simulink model "regulator_LQG_discrete_Ueq_comparison"  (R2019b)
settings: Solver=ode45  StartTime=0.0  StopTime=tsim  RelTol=1e-3  EnableMultiTasking=on
values from neighbouring files (symbols this model uses):
  B_noise = [B ones(size(B,1),1)]    [es3.m]
  C_states = eye(2)    [es3.m]
  D_noise = [D_states zeros(size(D_states,1),1)]    [es3.m]
  Klqr1 = dlqr(A,B,Q,R)    [es3.m]
  NK = 0    [es3.m]
  RK1 = 10*QK(1)    [es3.m]
  RK2 = QK(1)*0.1    [es3.m]
  sat_max = inf    [es3.m]
  sat_min = -inf    [es3.m]
  Ts = 0.1    [es3.m]
  Ubar = inv(dcgain(Gz))*Ybar    [es3.m]
  x0 = [5 20]    [es3.m]
  x0K = 1.5*x0    [es3.m]
  xref = Xbar    [es3.m]
undefined symbols (not defined in the file or in its folder): A, B, C, D, Discrete, Time
libraries: simulink x4, ctrlSharedLib x2
settings Model: Creator=Administrator  LastModifiedBy=Chiara
settings DataIOCC: LimitDataPoints=on  SaveFormat=Array  SignalLoggingSaveFormat=ModelDataLogs  ReturnWorkspaceOutputs=off
settings OptimizationCC: ExpressionDepthLimit=2147483647  InitFltsAndDblsToZero=on  LifeSpan=inf
settings DebuggingCC: UnderspecifiedInitializationDetection=Classic  MergeDetectMultiDrivingBlocksExec=none  SolverPrmCheckMsg=warning  FcnCallInpInsideContextMsg=warning  StateNameClashWarn=warning  SFUnexpectedBacktrackingDiag=warning  SFNoUnconditionalDefaultTransitionDiag=warning  SFExecutionAtInitializationDiag=none  ArithmeticOperatorsInVariantConditions=warning
settings HardwareCC: ProdBitPerPointer=32  ProdBitPerSizeT=32  ProdBitPerPtrDiffT=32  ProdLargestAtomicFloat=None  ProdIntDivRoundTo=Undefined  ProdEndianess=Unspecified  ProdWordSize=32  ProdHWDeviceType=32-bit Generic
settings ModelReferenceCC: PropagateSignalLabelsOutOfModel=off
settings SFSimCC: SimUseLocalCustomCode=off  CustomCodeUndefinedFunction=UseInterfaceOnly
settings RTWCC: RTWUseLocalCustomCode=off
settings CodeAppCC: StateflowObjectComments=on
settings GRTTargetCC: TargetLangStandard=C89/C90 (ANSI)  GeneratePreprocessorConditionals=Disable all  CombineOutputUpdateFcns=off  GRTInterface=on
settings ConfigComp: CovMetricSettings=dw  CovHtmlReporting=on  CovSaveCumulativeToWorkspaceVar=on  CovSaveSingleToWorkspaceVar=on  CovExternalEMLEnable=off  CovSFcnEnable=off

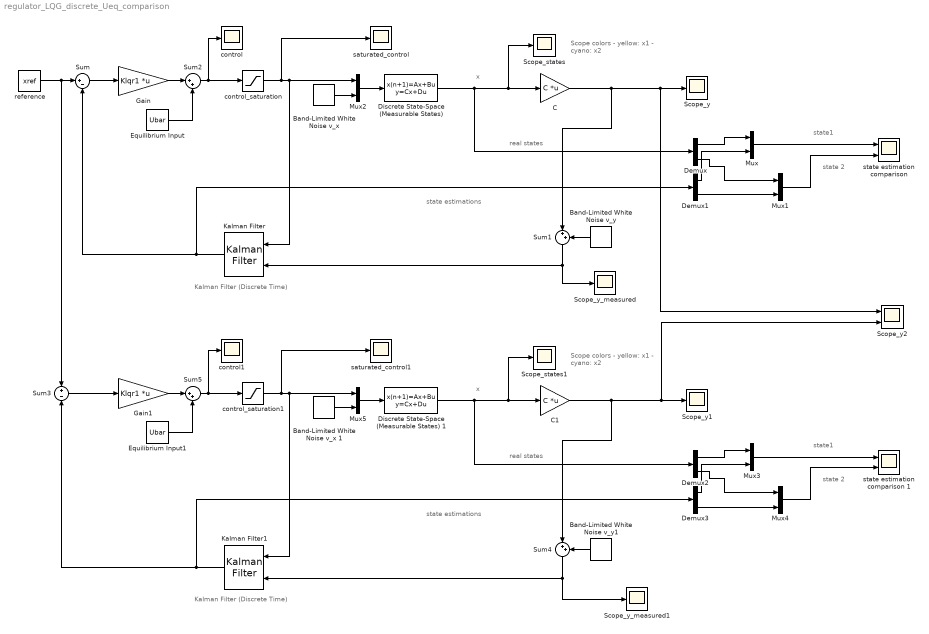
== system regulator_LQG_discrete_Ueq_comparison ==
  note: Kalman Filter (Discrete Time)
  note: state 2
  note: state1
  note: real states
  note: state estimations
  note: x
  note: Scope colors
      | - yellow: x1
      | - cyano: x2
  note: x
  note: state 2
  note: Scope colors
      | - yellow: x1
      | - cyano: x2
  note: Kalman Filter (Discrete Time)
  note: real states
  note: state1
  note: state estimations
  "Band-Limited White Noise v_x " : simulink/Sources/Band-Limited White Noise  Cov=power_vx1  Ts=Ts  seed=[23341]
  Band-Limited White Noise v_x 1 : simulink/Sources/Band-Limited White Noise  Cov=power_vx2  Ts=Ts  seed=[23341]
  Band-Limited White Noise v_y : simulink/Sources/Band-Limited White Noise  Cov=power_vy1  Ts=Ts  seed=[1258]
  Band-Limited White Noise v_y1 : simulink/Sources/Band-Limited White Noise  Cov=power_vy2  Ts=Ts  seed=[1258]
  C : Gain  Gain=C  Multiplication=Matrix(K*u)
  C1 : Gain  Gain=C  Multiplication=Matrix(K*u)
  Demux{,1..3} (4 alike) : Demux  Outputs=2
  "Discrete State-Space (Measurable States) " : DiscreteStateSpace  A=A  B=B_noise  C=C_states  D=D_noise  InitialCondition=x0  SampleTime=Ts
  Discrete State-Space (Measurable States) 1 : DiscreteStateSpace  A=A  B=B_noise  C=C_states  D=D_noise  InitialCondition=x0  SampleTime=Ts
  Equilibrium Input : Constant  Value=Ubar
  Equilibrium Input1 : Constant  Value=Ubar
  Gain : Gain  Gain=Klqr1  Multiplication=Matrix(K*u)
  Gain1 : Gain  Gain=Klqr1  Multiplication=Matrix(K*u)
  Kalman Filter : ctrlSharedLib/Kalman Filter  TimeDomain=Discrete-Time  UseCurrentEstimator=on  ModelSource=Individual A, B, C, D matrices  ModelSourceVariable=ss(0.95,1,1,0,1)  A=A  B=B  C=C  D=D  NumberOfStates=1  NumberOfInputs=1  NumberOfOutputs=1  InitialEstimateSource=Dialog  X0=x0K  P0=10  UseK=off  UseGH=off  NumberOfProcessNoiseInputs=1  G=1  TimeInvariantG=on  H=0  TimeInvariantH=on  Q=QK  TimeInvariantQ=on  R=RK1  TimeInvariantR=on  N=NK  TimeInvariantN=on  AddInputPort=on  AddEnablePort=off  OutputEstimatedY=off  OutputP=off  Ts=Ts
      settings: SourceProductBaseCode=CT
  Kalman Filter1 : ctrlSharedLib/Kalman Filter  TimeDomain=Discrete-Time  UseCurrentEstimator=on  ModelSource=Individual A, B, C, D matrices  ModelSourceVariable=ss(0.95,1,1,0,1)  A=A  B=B  C=C  D=D  NumberOfStates=1  NumberOfInputs=1  NumberOfOutputs=1  InitialEstimateSource=Dialog  X0=x0K  P0=10  UseK=off  UseGH=off  NumberOfProcessNoiseInputs=1  G=1  TimeInvariantG=on  H=0  TimeInvariantH=on  Q=QK  TimeInvariantQ=on  R=RK2  TimeInvariantR=on  N=NK  TimeInvariantN=on  AddInputPort=on  AddEnablePort=off  OutputEstimatedY=off  OutputP=off  Ts=Ts
      settings: SourceProductBaseCode=CT
  Mux{,1..5} (6 alike) : Mux  Inputs=2
  Scope_states : Scope
  Scope_states1 : Scope
  Scope_y : Scope
  Scope_y1 : Scope
  Scope_y2 : Scope  NumInputPorts=2
  Scope_y_measured : Scope
  Scope_y_measured1 : Scope
  Sum : Sum  Inputs=|+-
  Sum{1..2,4..5} (4 alike) : Sum  Inputs=|++
  Sum3 : Sum  Inputs=+-
  control : Scope
  control1 : Scope
  control_saturation : Saturate  UpperLimit=sat_max  LowerLimit=sat_min
  control_saturation1 : Saturate  UpperLimit=sat_max  LowerLimit=sat_min
  reference : Constant  Value=xref
  saturated_control : Scope
  saturated_control1 : Scope
  "state estimation comparison " : Scope  NumInputPorts=2
  state estimation comparison 1 : Scope  NumInputPorts=2
  wires:
  reference/1 -> Sum3/1, Sum/1
  Sum/1 -> Gain/1
  "Discrete State-Space (Measurable States) "/1 -> Demux/1, Scope_states/1, C/1
  C/1 -> Sum1/1, Scope_y/1, Scope_y2/1
  control_saturation/1 -> Mux2/1, Kalman Filter/1, saturated_control/1
  Demux/1 -> Mux/1
  Demux1/1 -> Mux/2
  Demux1/2 -> Mux1/2
  Demux/2 -> Mux1/1
  Mux1/1 -> "state estimation comparison "/2
  Mux/1 -> "state estimation comparison "/1
  Mux2/1 -> "Discrete State-Space (Measurable States) "/1
  Sum1/1 -> Scope_y_measured/1, Kalman Filter/2
  Band-Limited White Noise v_y/1 -> Sum1/2
  "Band-Limited White Noise v_x "/1 -> Mux2/2
  Gain/1 -> Sum2/1
  Sum2/1 -> control/1, control_saturation/1
  Equilibrium Input/1 -> Sum2/2
  Demux3/1 -> Mux3/2
  Gain1/1 -> Sum5/1
  Sum3/1 -> Gain1/1
  Demux2/1 -> Mux3/1
  Sum5/1 -> control1/1, control_saturation1/1
  Equilibrium Input1/1 -> Sum5/2
  Sum4/1 -> Scope_y_measured1/1, Kalman Filter1/2
  Demux2/2 -> Mux4/1
  Mux4/1 -> state estimation comparison 1/2
  Mux3/1 -> state estimation comparison 1/1
  Band-Limited White Noise v_x 1/1 -> Mux5/2
  Kalman Filter1/1 -> Demux3/1, Sum3/2
  C1/1 -> Sum4/1, Scope_y1/1, Scope_y2/2
  Band-Limited White Noise v_y1/1 -> Sum4/2
  Mux5/1 -> Discrete State-Space (Measurable States) 1/1
  Discrete State-Space (Measurable States) 1/1 -> Demux2/1, Scope_states1/1, C1/1
  Demux3/2 -> Mux4/2
  Kalman Filter/1 -> Demux1/1, Sum/2
  control_saturation1/1 -> Mux5/1, Kalman Filter1/1, saturated_control1/1
